simulink model "modeltest"  (Simulink 8.5)
settings: Solver=ode45  StartTime=0.0  StopTime=10.0  RelTol=1e-3
values from neighbouring files (symbols this model uses):
  Pmax = 20000    [modeltest.m]
settings Model: Creator=nogueira_raf  LastModifiedBy=nogueira_raf
settings DataIOCC: SignalLoggingSaveFormat=Dataset
settings OptimizationCC: ExpressionDepthLimit=128
settings DebuggingCC: UnderspecifiedInitializationDetection=Simplified  MergeDetectMultiDrivingBlocksExec=error  FcnCallInpInsideContextMsg=EnableAllAsError  StateNameClashWarn=none
settings GRTTargetCC: CombineOutputUpdateFcns=on  GRTInterface=off

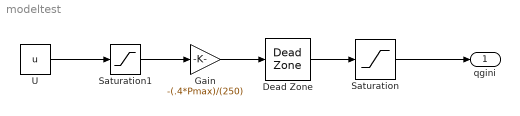
== system modeltest ==
  Dead Zone : DeadZone  LowerValue=19250  UpperValue=20750  SaturateOnIntegerOverflow=on
  Gain : Gain  Gain=-(.4*Pmax)/(250)
  Saturation : Saturate  UpperLimit=0.4*Pmax  LowerLimit=-0.4*Pmax
  Saturation1 : Saturate  UpperLimit=21000  LowerLimit=18000
  U : Constant  Value=u
  qgini : Outport
  wires:
  U/1 -> Saturation1/1
  Saturation/1 -> qgini/1
  Dead Zone/1 -> Saturation/1
  Gain/1 -> Dead Zone/1
  Saturation1/1 -> Gain/1
